simulink model "Regelung_V3"  (R2021b)
settings: Solver=VariableStepAuto  StartTime=0.0  StopTime=10.0  RelTol=1e-3  EnableMultiTasking=on
values from neighbouring files (symbols this model uses):
  M_AP = double(M_AP)    [linearisierung.m]
undefined symbols (not defined in the file or in its folder): AP, K, stObs, stPendel, x0
settings Model: Creator=gong  LastModifiedBy=caio
settings SolverCC: AlgebraicLoopSolver=TrustRegion
settings DataIOCC: LimitDataPoints=on  SaveFormat=Array  ReturnWorkspaceOutputs=off
settings OptimizationCC: LifeSpan=inf
settings DebuggingCC: SFUnexpectedBacktrackingDiag=warning  SFNoUnconditionalDefaultTransitionDiag=warning  SFMachineParentedDataDiag=warning  ArithmeticOperatorsInVariantConditions=warning
settings HardwareCC: ProdBitPerPointer=32  ProdBitPerSizeT=32  ProdBitPerPtrDiffT=32  ProdLargestAtomicFloat=None  ProdIntDivRoundTo=Undefined  ProdEndianess=Unspecified  ProdWordSize=32  ProdHWDeviceType=32-bit Generic
settings ModelReferenceCC: PropagateSignalLabelsOutOfModel=off
settings SFSimCC: SimUseLocalCustomCode=off  CustomCodeUndefinedFunction=UseInterfaceOnly
settings RTWCC: RTWUseLocalCustomCode=off
settings CodeAppCC: StateflowObjectComments=on
settings GRTTargetCC: TargetLangStandard=C89/C90 (ANSI)
settings ConfigComp: CovMetricSettings=dw  CovSaveCumulativeToWorkspaceVar=on  CovSaveSingleToWorkspaceVar=on  CovExternalEMLEnable=off

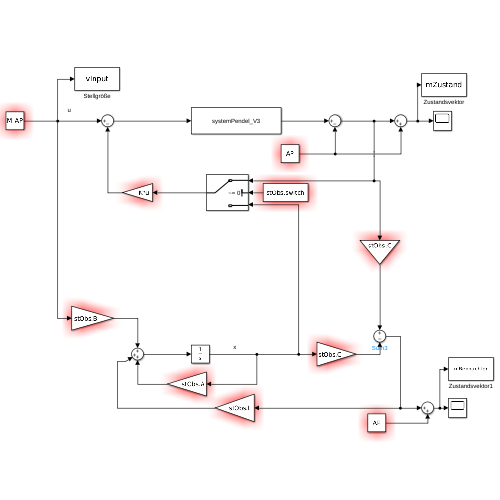
[thumbnail: Simulink's stored preview of the top-level diagram]
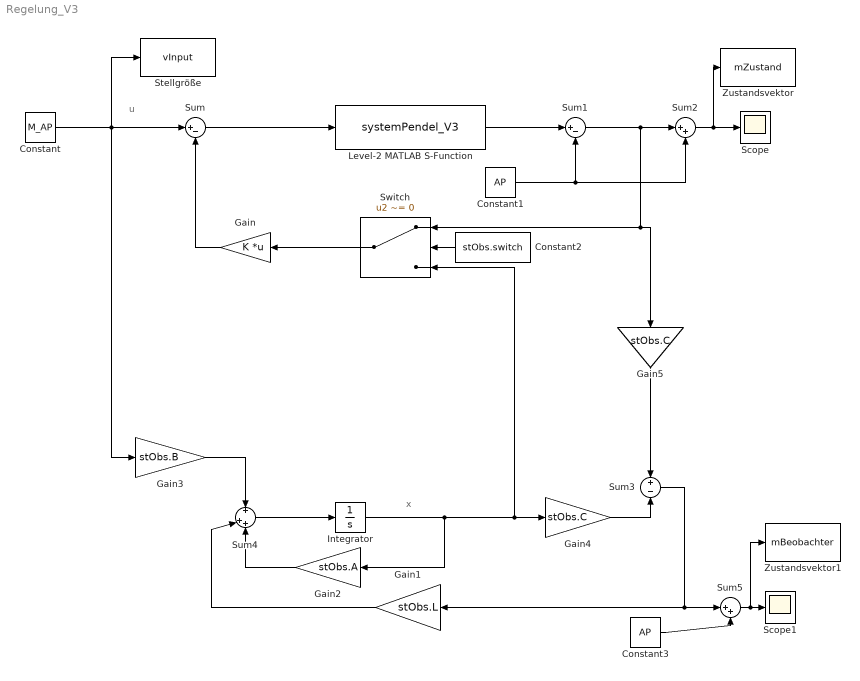
== system Regelung_V3 ==
  note: u
  note: x
  Constant : Constant  Value=M_AP
  Constant1 : Constant  Value=AP
  Constant2 : Constant  Value=stObs.switch
  Constant3 : Constant  Value=AP
  Gain : Gain  Gain=K  Multiplication=Matrix(K*u)
  Gain1 : Gain  Gain=stObs.L
  Gain2 : Gain  Gain=stObs.A
  Gain3 : Gain  Gain=stObs.B
  Gain4 : Gain  Gain=stObs.C
  Gain5 : Gain  Gain=stObs.C
  Integrator : Integrator
  Level-2 MATLAB S-Function : M-S-Function  FunctionName=systemPendel_V3  Parameters=stPendel,x0
  Scope : Scope
  Scope1 : Scope
  Stellgröße : ToWorkspace  VariableName=vInput  SaveFormat=Timeseries  SampleTime=-1
  Sum : Sum  Inputs=|+-
  Sum1 : Sum  Inputs=|+-
  Sum2 : Sum  Inputs=|++
  Sum3 : Sum  Inputs=+|-
  Sum4 : Sum  Inputs=+|++
  Sum5 : Sum  Inputs=|++
  Switch : Switch  Criteria=u2 ~= 0
  Zustandsvektor : ToWorkspace  VariableName=mZustand  SaveFormat=Timeseries  SampleTime=-1
  Zustandsvektor1 : ToWorkspace  VariableName=mBeobachter  SaveFormat=Timeseries  SampleTime=-1
  wires:
  Gain/1 -> Sum/2
  Constant/1 -> Gain3/1, Stellgröße/1, Sum/1
  Sum/1 -> Level-2 MATLAB S-Function/1
  Level-2 MATLAB S-Function/1 -> Sum1/1
  Sum1/1 -> Gain5/1, Switch/1, Sum2/1
  Constant1/1 -> Sum2/2, Sum1/2
  Sum2/1 -> Zustandsvektor/1, Scope/1
  Sum3/1 -> Sum5/1, Gain1/1
  Sum4/1 -> Integrator/1
  Gain3/1 -> Sum4/1
  Gain1/1 -> Sum4/2
  Gain4/1 -> Sum3/2
  Integrator/1 -> Switch/3, Gain4/1, Gain2/1
  Switch/1 -> Gain/1
  Constant2/1 -> Switch/2
  Gain5/1 -> Sum3/1
  Gain2/1 -> Sum4/3
  Constant3/1 -> Sum5/2
  Sum5/1 -> Zustandsvektor1/1, Scope1/1
